simulink model "KeyEventGeneratorReplacementRefMod"  (R2016b)
settings: Solver=VariableStepAuto  StartTime=0.0  StopTime=10.0  RelTol=1e-3
undefined symbols (not defined in the file or in its folder): selection
settings Model: DataDictionary=DataDictionary.sldd  Creator=Taeke  LastModifiedBy=lucadelaat

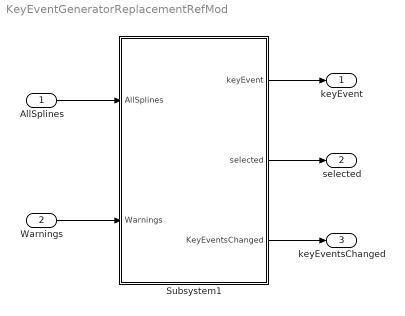
== system KeyEventGeneratorReplacementRefMod ==
  AllSplines : Inport
  Warnings : Inport  Port=2
  Subsystem1 : Subsystem
  keyEvent : Outport  OutDataTypeStr=Bus: keyEventTotal
  selected : Outport  Port=2
  keyEventsChanged : Outport  Port=3
  wires:
  AllSplines/1 -> Subsystem1/1(AllSplines)
  Warnings/1 -> Subsystem1/2(Warnings)
  Subsystem1/1(keyEvent) -> keyEvent/1
  Subsystem1/2(selected) -> selected/1
  Subsystem1/3(KeyEventsChanged) -> keyEventsChanged/1

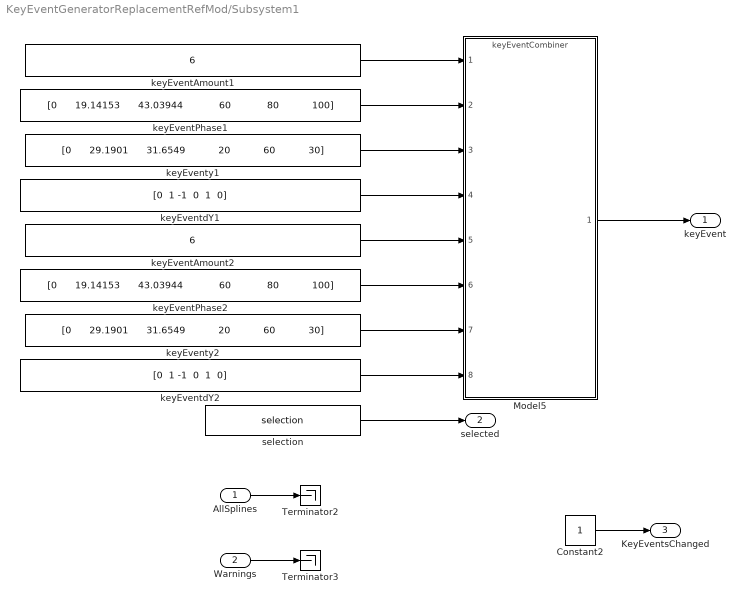
== system KeyEventGeneratorReplacementRefMod/Subsystem1 ==
  AllSplines : Inport
  Warnings : Inport  Port=2
  Constant2 : Constant
  Model5 : ModelReference  ModelNameDialog=keyEventCombiner.slx  SimulationMode=Normal  ModelReferenceVersion=1.6
  Terminator2 : Terminator
  Terminator3 : Terminator
  keyEventAmount1 : Constant  Value=6
  keyEventAmount2 : Constant  Value=6
  keyEventPhase1 : Constant  Value="[0      19.14153      43.03944            60            80           100]"
  keyEventPhase2 : Constant  Value="[0      19.14153      43.03944            60            80           100]"
  keyEventdY1 : Constant  Value="[0  1 -1  0  1  0]"
  keyEventdY2 : Constant  Value="[0  1 -1  0  1  0]"
  keyEventy1 : Constant  Value="[0      29.1901      31.6549           20           60           30]"
  keyEventy2 : Constant  Value="[0      29.1901      31.6549           20           60           30]"
  selection : Constant  Value=selection
  keyEvent : Outport
  selected : Outport  Port=2
  KeyEventsChanged : Outport  Port=3
  wires:
  Warnings/1 -> Terminator3/1
  keyEventdY2/1 -> Model5/8
  AllSplines/1 -> Terminator2/1
  keyEventy1/1 -> Model5/3
  Constant2/1 -> KeyEventsChanged/1
  keyEventdY1/1 -> Model5/4
  keyEventPhase1/1 -> Model5/2
  keyEventPhase2/1 -> Model5/6
  keyEventAmount1/1 -> Model5/1
  keyEventy2/1 -> Model5/7
  Model5/1 -> keyEvent/1
  keyEventAmount2/1 -> Model5/5
  selection/1 -> selected/1
